simulink model "ProcessModel"  (R2019b)
settings: Solver=VariableStepAuto  StartTime=0.0  StopTime=10.0  RelTol=1e-3
settings Model: Creator=Daniel  LastModifiedBy=Daniel

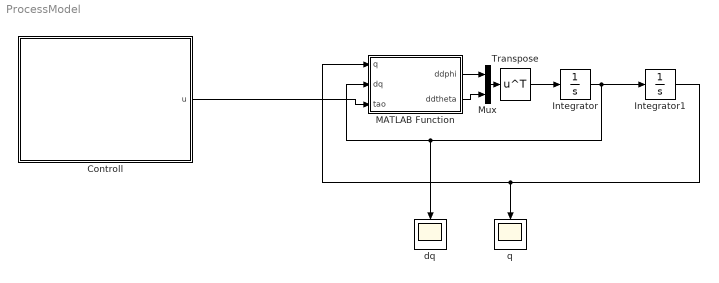
== system ProcessModel ==
  Controll : Subsystem
  Integrator : Integrator
  Integrator1 : Integrator
  MATLAB Function : MATLAB Function  TreatAsAtomicUnit=on
  Mux : Mux  Inputs=2
  Transpose : Math  Operator=transpose  SignedPower=off  SaturateOnIntegerOverflow=on
  dq : Scope
  q : Scope
  wires:
  Integrator/1 -> MATLAB Function/2(dq), dq/1, Integrator1/1
  Integrator1/1 -> MATLAB Function/1(q), q/1
  Controll/1(u) -> MATLAB Function/3(tao)
  MATLAB Function/1(ddphi) -> Mux/1
  MATLAB Function/2(ddtheta) -> Mux/2
  Mux/1 -> Transpose/1
  Transpose/1 -> Integrator/1

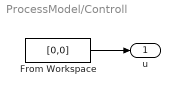
== system ProcessModel/Controll ==
  From Workspace : FromWorkspace  VariableName=[0,0]  SampleTime=0
  u : Outport
  wires:
  From Workspace/1 -> u/1

== matlab function ProcessModel/MATLAB Function ==
  data: q input; ddphi output; dq input; tao input; ddtheta output
function [ddphi, ddtheta] = fcn(q,dq,tao)
x=[q;dq];
%% x= [phi, theta, dphi, dtheta] i process lineariserat kring x0=(0,0,0,0)
denum= alpha*beta - gamma^2;

A=[0,1,0,0; 0,0,0,1; 
    0,0, -((delta*gamma)/(denum)), 0; 0,0, ((alpha*delta)/(denum)),0];
B=[0,0; 0,0; ((beta)/(denum)), -((gamma)/(denum)) ; -(gamma/(denum)), (alpha/(denum))];
C=[0,0,1,0;
    0,0,0,1];
D=[0,0;
    0,0];

dx = A*x + B*tao
ddq = C*dx + D*tao;
ddphi = ddq(1,1);
ddtheta = ddq(2,1);
end
